simulink model "sim"  (R2026a)
settings: Solver=FixedStepDiscrete  StopTime=150  FixedStep=0.01  EnableMultiTasking=on
InitFcn:
  | % run MPC\MPC_2_Parameters.m
  | Ts = 1;
undefined symbols (not defined in the file): DiscIntNeverNeededParam
libraries: simulink x1
settings Model: SimulationMode=external  Creator=danis  LastModifiedBy=danis
settings SolverCC: ConcurrentTasks=on  PositivePriorityOrder=on  InsertRTBMode=Never (minimum delay)
settings DataIOCC: SaveState=on  SignalLoggingName=logsOut
settings OptimizationCC: BooleanDataType=off  OptimizeBlockIOStorage=off  BufferReuse=off  GlobalBufferReuse=off  ExpressionFolding=off  LocalBlockOutputs=off  InitFltsAndDblsToZero=on  OptimizeDataStoreBuffers=off  BusAssignmentInplaceUpdate=off
settings DebuggingCC: SaveWithParameterizedLinksMsg=none  UnderspecifiedInitializationDetection=Classic  CheckExecutionContextPreStartOutputMsg=on  SignalResolutionControl=TryResolveAllWithWarning  TasksWithSamePriorityMsg=none
settings HardwareCC: ProdBitPerLong=64.0  ProdHWDeviceType=Intel->x86-64 (Linux 64)
settings SFSimCC: SimTargetLang=C++
settings RTWCC: BuildConfiguration=Faster Runs
settings ConfigComp: PLC_TargetIDE=generic  PLC_MultiTBSigbuilderTimeRange=off  PLC_FoldFBCallOutputVar=off  PLC_RemoveUnusedSSMethodCallArguments=off  PLC_UseCallOutputArgSyntax=off  PLC_EnableUnsignedAndDoubleTypes=off  PLC_EnableUDTSplitting=off  PLC_MaxFieldsInUDT=500.0  PLC_InlineEnumCastFunction=off  PLC_RTWMaxIdLength=31.0  PLC_RollThreshold=5.0  PLC_ActiveTab=0.0  PLC_EnableStringLiteralTB=on  PLC_Enable64bitIntSupport=off

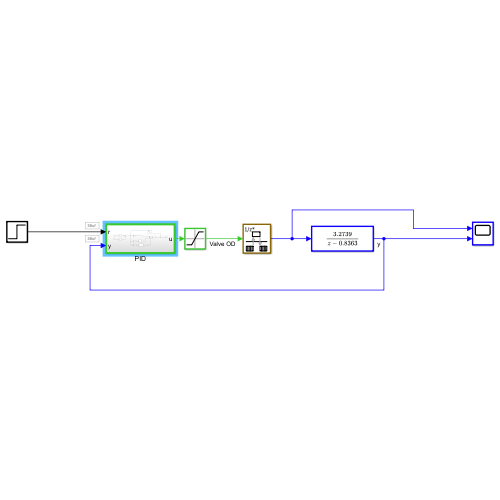
[thumbnail: Simulink's stored preview of the top-level diagram]
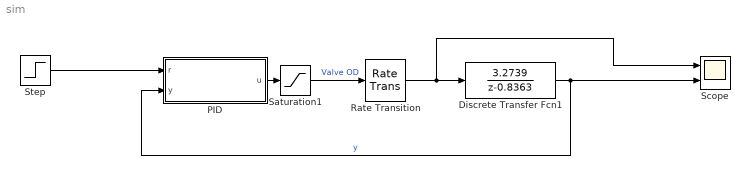
== system sim ==
  Discrete Transfer Fcn1 : DiscreteTransferFcn  Numerator=[3.2739]  Denominator="[1  -0.8363]"
  PID : Subsystem  TreatAsAtomicUnit=on  SystemSampleTime=0.02
  Rate Transition : RateTransition  OutPortSampleTime=1
  Saturation1 : Saturate  UpperLimit=0.9  LowerLimit=0.1
  Scope : Scope  NumInputPorts=2
      settings: ActiveDisplayYMinimum=-1.9508779531657583  ActiveDisplayYMaximum=17.55790157849183  DataLoggingVariableName=ScopeData2
  Step : Step  Time=50  InitialValue=8  FinalValue=13  SampleTime=0
  wires:
  Saturation1/1 -> Rate Transition/1  "Valve OD"
  Step/1 -> PID/1(r)
  PID/1(u) -> Saturation1/1
  Discrete Transfer Fcn1/1 -> PID/2(y), Scope/2  "y"
  Rate Transition/1 -> Scope/1, Discrete Transfer Fcn1/1

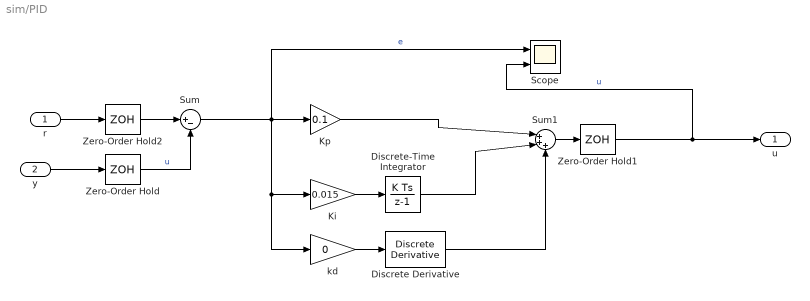
== system sim/PID ==
  r : Inport
  y : Inport  Port=2
  Discrete Derivative : simulink/Discrete/Discrete Derivative  gainval=1.0  ICPrevScaledInput=0.0  OutMin=[]  OutMax=[]  OutDataType=fixdt(1, 16)  OutScaling=2^-10  DoSatur=off
  Discrete-Time Integrator : DiscreteIntegrator  SampleTime=-1  ICPrevOutput=DiscIntNeverNeededParam  ICPrevScaledInput=DiscIntNeverNeededParam
  Ki : Gain  Gain=0.015
  Kp : Gain  Gain=0.1
  Scope : Scope  NumInputPorts=2
      settings: ActiveDisplayYMinimum=-5.4109752682555126  ActiveDisplayYMaximum=10.643099708129036
  Sum : Sum  Inputs=|+-
  Sum1 : Sum  Inputs=|+++
  Zero-Order Hold : ZeroOrderHold  SampleTime=-1
  Zero-Order Hold1 : ZeroOrderHold  SampleTime=-1
  Zero-Order Hold2 : ZeroOrderHold  SampleTime=-1
  kd : Gain  Gain=0
  u : Outport
  wires:
  r/1 -> Zero-Order Hold2/1
  y/1 -> Zero-Order Hold/1
  Sum/1 -> Scope/1, Ki/1, kd/1, Kp/1  "e"
  Ki/1 -> Discrete-Time Integrator/1
  kd/1 -> Discrete Derivative/1
  Kp/1 -> Sum1/1
  Discrete-Time Integrator/1 -> Sum1/2
  Discrete Derivative/1 -> Sum1/3
  Sum1/1 -> Zero-Order Hold1/1
  Zero-Order Hold1/1 -> u/1, Scope/2  "u"
  Zero-Order Hold2/1 -> Sum/1
  Zero-Order Hold/1 -> Sum/2  "u"
